simulink model "cic_dezim_1_"  (Simulink 7.8)
settings: Solver=FixedStepDiscrete  SolverMode=SingleTasking  StartTime=0.0  StopTime=10.0  FixedStep=1e-5  RelTol=1e-3
values from neighbouring files (symbols this model uses):
  Hm = mfilt.cicdecim(R,M,N)    [cic_dezim1.m]    (also in cic_dezim1_.m; cic_dezim2.m)
  hpfir = fir1(nord, 0.1*2)    [cic_dezim1_.m]
libraries: dspsigops x1
settings Model: Creator=svenhoffmann  LastModifiedBy=josef  ExtModeAutoUpdateStatusClock=off
settings OptimizationCC: InlineInvariantSignals=on  InitFltsAndDblsToZero=on
settings DebuggingCC: SaveWithParameterizedLinksMsg=none  SignalResolutionControl=TryResolveAllWithWarning  MultiTaskDSMMsg=warning  MultiTaskCondExecSysMsg=none  StrictBusMsg=None
settings RTWCC: IncludeERTFirstTime=on
settings GRTTargetCC: TargetFcnLib=ansi_tfl_tmw.mat

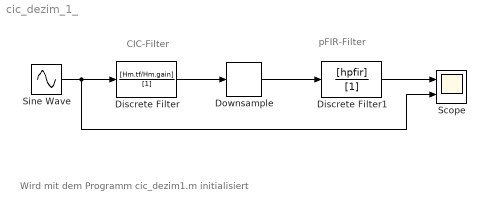
== system cic_dezim_1_ ==
  note: CIC-Filter
  note: Wird mit dem Programm cic_dezim1.m
      | initialisiert
  note: pFIR-Filter
  Discrete Filter : DiscreteFilter  Numerator=[Hm.tf/Hm.gain]  Denominator=[1]
  Discrete Filter1 : DiscreteFilter  Numerator=[hpfir]  Denominator=[1]
  Downsample : dspsigops/Downsample  N=8  phase=0  InputProcessing=Inherited (this choice will be removed - see release notes)  RateOptions=Enforce single-rate processing  smode=Allow multirate  fmode=Maintain input frame size  ic=0
  Scope : Scope  NumInputPorts=2
      settings: YMin=-5~-5  YMax=5~5
  Sine Wave : Sin  Frequency=2*pi*210  SampleTime=1/1000
  wires:
  Sine Wave/1 -> Discrete Filter/1, Scope/2
  Discrete Filter/1 -> Downsample/1
  Downsample/1 -> Discrete Filter1/1
  Discrete Filter1/1 -> Scope/1
